simulink model "Frec_Nat_s_mk"  (R2020a)
settings: Solver=ode4  StartTime=0.0  StopTime=10  FixedStep=0.001  RelTol=1e-3
values from neighbouring files (symbols this model uses):
  F = [200    300     400       500     600    700     800     900 1000 1100 1200]    [k.m]    (also in wn.m = P3*e*w^2)
  k1 = k*E*I/(a^3)    [wn.m]
  Mt1 = M+m    [wn.m]
  w = rpm/60    [wn.m]
settings Model: Creator=karli  LastModifiedBy=karli

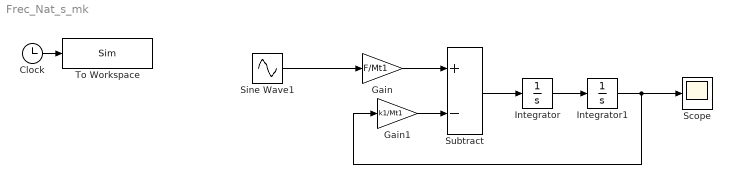
== system Frec_Nat_s_mk ==
  Clock : Clock
  Gain : Gain  Gain=F/Mt1
  Gain1 : Gain  Gain=k1/Mt1
  Integrator : Integrator
  Integrator1 : Integrator
  Scope : Scope
  Sine Wave1 : Sin  Amplitude=F  Frequency=w  SampleTime=0
  Subtract : Sum  Inputs=+-
  To Workspace : ToWorkspace  VariableName=Sim  SampleTime=-1
  wires:
  Clock/1 -> To Workspace/1
  Integrator/1 -> Integrator1/1
  Integrator1/1 -> Gain1/1, Scope/1
  Gain/1 -> Subtract/1
  Gain1/1 -> Subtract/2
  Subtract/1 -> Integrator/1
  Sine Wave1/1 -> Gain/1
